simulink model "aircraft_pitch_lqr_multibody"  (R2022b)
settings: Solver=ode23t  StartTime=0.0  StopTime=stopTime  MaxStep=0.005  RelTol=1e-9  AbsTol=1e-11
model workspace (MAT data in the model file):
  Jpitch = 1
  K = [-0.5605 76.158 2.1817]
  Ki = 0
  Nbar = 2.1817
  aScale = 1
  biasAcceleration = 0
  biasStartTime = 30
  biasTime = 20
  deltaMax = 0.436332312999
  elevatorBias = 0
  geometryInertia = 4.77572166667
  integratorThreshold = 0.0174532925199
  massScale = 1
  r = 0.2
  stopTime = 30
undefined symbols (not defined in the file or in its folder): X, Y, Z
libraries: sm_lib x9, nesl_utility x4
settings Model: Creator=shark  LastModifiedBy=shark

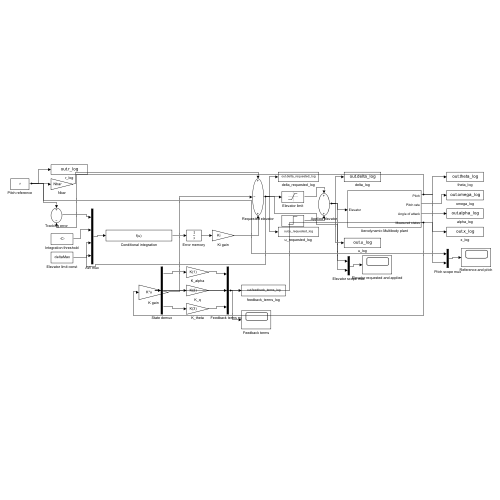
[thumbnail: Simulink's stored preview of the top-level diagram]
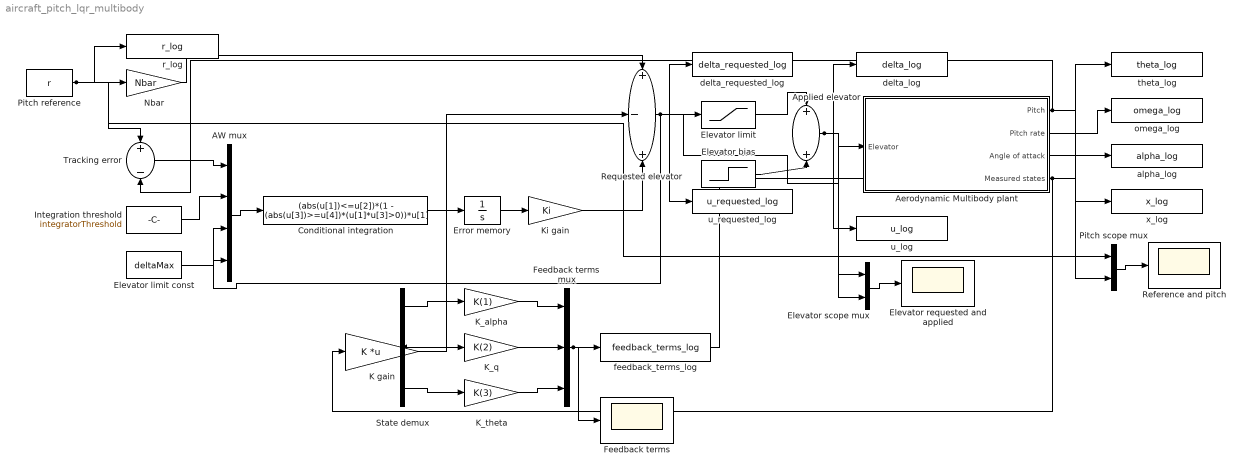
== system aircraft_pitch_lqr_multibody ==
  AW mux : Mux
  Aerodynamic Multibody plant : Subsystem
  Applied elevator : Sum
  Conditional integration : Fcn  Expr=(abs(u[1])<=u[2])*(1 - (abs(u[3])>=u[4])*(u[1]*u[3]>0))*u[1]
  Elevator bias : Step  Time=biasStartTime  After=elevatorBias  SampleTime=0
  Elevator limit : Saturate  UpperLimit=deltaMax  LowerLimit=-deltaMax
  Elevator limit const : Constant  Value=deltaMax
  Elevator requested and applied : Scope
  Elevator scope mux : Mux  Inputs=2
  Error memory : Integrator
  Feedback terms : Scope
  Feedback terms mux : Mux  Inputs=3
  Integration threshold : Constant  Value=integratorThreshold
  K gain : Gain  Gain=K  Multiplication=Matrix(K*u)
  K_alpha : Gain  Gain=K(1)
  K_q : Gain  Gain=K(2)
  K_theta : Gain  Gain=K(3)
  Ki gain : Gain  Gain=Ki
  Nbar : Gain  Gain=Nbar
  Pitch reference : Constant  Value=r
  Pitch scope mux : Mux  Inputs=2
  Reference and pitch : Scope
  Requested elevator : Sum  Inputs=+-+
  State demux : Demux  Outputs=3
  Tracking error : Sum  Inputs=+-
  alpha_log : ToWorkspace  VariableName=alpha_log  SaveFormat=Timeseries  SampleTime=-1
  delta_log : ToWorkspace  VariableName=delta_log  SaveFormat=Timeseries  SampleTime=-1
  delta_requested_log : ToWorkspace  VariableName=delta_requested_log  SaveFormat=Timeseries  SampleTime=-1
  feedback_terms_log : ToWorkspace  VariableName=feedback_terms_log  SaveFormat=Timeseries  SampleTime=-1
  omega_log : ToWorkspace  VariableName=omega_log  SaveFormat=Timeseries  SampleTime=-1
  r_log : ToWorkspace  VariableName=r_log  SaveFormat=Timeseries  SampleTime=-1
  theta_log : ToWorkspace  VariableName=theta_log  SaveFormat=Timeseries  SampleTime=-1
  u_log : ToWorkspace  VariableName=u_log  SaveFormat=Timeseries  SampleTime=-1
  u_requested_log : ToWorkspace  VariableName=u_requested_log  SaveFormat=Timeseries  SampleTime=-1
  x_log : ToWorkspace  VariableName=x_log  SaveFormat=Timeseries  SampleTime=-1
  wires:
  Pitch reference/1 -> Nbar/1, Tracking error/1, r_log/1, Pitch scope mux/1
  Aerodynamic Multibody plant/1(Pitch) -> Tracking error/2, theta_log/1, Pitch scope mux/2
  Tracking error/1 -> AW mux/1
  Integration threshold/1 -> AW mux/2
  Requested elevator/1 -> AW mux/3, Elevator limit/1, delta_requested_log/1, u_requested_log/1, Elevator scope mux/1
  Elevator limit const/1 -> AW mux/4
  AW mux/1 -> Conditional integration/1
  Conditional integration/1 -> Error memory/1
  Error memory/1 -> Ki gain/1
  Aerodynamic Multibody plant/4(Measured states) -> K gain/1, State demux/1, x_log/1
  State demux/1 -> K_alpha/1
  State demux/2 -> K_q/1
  State demux/3 -> K_theta/1
  K_alpha/1 -> Feedback terms mux/1
  K_q/1 -> Feedback terms mux/2
  K_theta/1 -> Feedback terms mux/3
  Nbar/1 -> Requested elevator/1
  K gain/1 -> Requested elevator/2
  Ki gain/1 -> Requested elevator/3
  Elevator limit/1 -> Applied elevator/1
  Elevator bias/1 -> Applied elevator/2
  Applied elevator/1 -> Aerodynamic Multibody plant/1(Elevator), delta_log/1, u_log/1, Elevator scope mux/2
  Aerodynamic Multibody plant/2(Pitch rate) -> omega_log/1
  Aerodynamic Multibody plant/3(Angle of attack) -> alpha_log/1
  Feedback terms mux/1 -> feedback_terms_log/1, Feedback terms/1
  Pitch scope mux/1 -> Reference and pitch/1
  Elevator scope mux/1 -> Elevator requested and applied/1

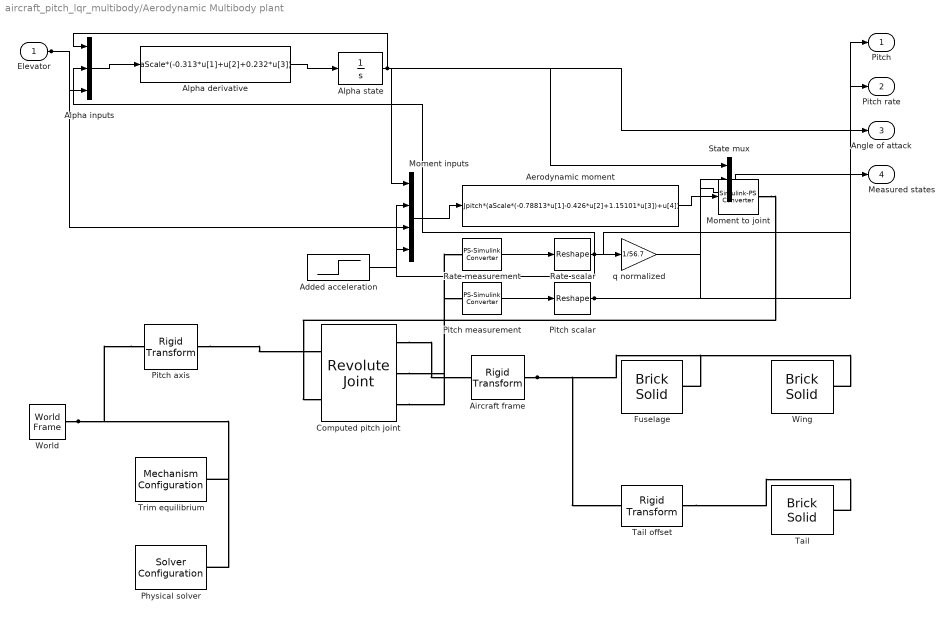
== system aircraft_pitch_lqr_multibody/Aerodynamic Multibody plant ==
  Elevator : Inport
  Added acceleration : Step  Time=biasTime  After=biasAcceleration  SampleTime=0
  Aerodynamic moment : Fcn  Expr=Jpitch*(aScale*(-0.78813*u[1]-0.426*u[2]+1.15101*u[3])+u[4])
  Aircraft frame : sm_lib/Frames and Transforms/Rigid Transform  TranslationMethod=None  TranslationStandardOffset=0  TranslationLengthUnit=m  TranslationStandardAxis=+Z  TranslationCartesianOffset=[0 0 0]  TranslationROffset=0  TranslationROffsetUnits=m  TranslationZOffset=0  TranslationZOffsetUnits=m  TranslationThetaOffset=0  TranslationThetaOffsetUnits=deg  RotationMethod=StandardAxis  RotationAngleUnits=deg  RotationStandardAxis=+X  RotationAngle=-90  RotationArbitraryAxis=[0 0 1]  FollAlignAxisA=+X  BaseAlignAxisA=+Y  FollAlignAxisB=+Y  BaseAlignAxisB=+Z  RotationSequenceAxes=FollowerAxes  RotationSequence=XYX  RotationSequenceAngles=[0 0 0]  RotationSequenceAnglesUnits=deg  RotationMatrix=[1 0 0; 0 1 0; 0 0 1]  Quaternion=[1 0 0 0]
  Alpha derivative : Fcn  Expr=aScale*(-0.313*u[1]+u[2]+0.232*u[3])
  Alpha inputs : Mux  Inputs=3
  Alpha state : Integrator
  Computed pitch joint : sm_lib/Joints/Revolute Joint  JointMode=Normal  SenseConstraintForce=off  SenseConstraintForceX=off  SenseConstraintForceY=off  SenseConstraintForceZ=off  SenseConstraintTorque=off  SenseConstraintTorqueX=off  SenseConstraintTorqueY=off  SenseConstraintTorqueZ=off  SenseTotalForce=off  SenseTotalForceX=off  SenseTotalForceY=off  SenseTotalForceZ=off  SenseTotalTorque=off  SenseTotalTorqueX=off  SenseTotalTorqueY=off  SenseTotalTorqueZ=off  CompositeWrenchDir=FollowerOnBase  CompositeWrenchFrame=BaseFrame  EquilibriumPosition=0  EquilibriumPositionUnits=deg  SpringStiffness=0  SpringStiffnessUnits=N*m/deg  DampingCoefficient=0  DampingCoefficientUnits=N*m/(deg/s)  TorqueActuationMode=InputTorque  MotionActuationMode=ComputedMotion  SensePosition=on  SenseVelocity=on  SenseAcceleration=off  SenseTorqueForce=off  SenseLowerLimitTorqueForce=off  SenseUpperLimitTorqueForce=off  LowerLimitSpecify=off  LowerLimitBound=-90  LowerLimitBoundUnits=deg  LowerLimitStiffness=1e4  LowerLimitStiffnessUnits=N*m/deg  LowerLimitDamping=10  LowerLimitDampingUnits=N*m/(deg/s)  LowerLimitTransitionRegionWidth=0.1  LowerLimitTransitionRegionWidthUnits=deg  UpperLimitSpecify=off  UpperLimitBound=90  UpperLimitBoundUnits=deg  UpperLimitStiffness=1e4  UpperLimitStiffnessUnits=N*m/deg  UpperLimitDamping=10  UpperLimitDampingUnits=N*m/(deg/s)  UpperLimitTransitionRegionWidth=0.1  UpperLimitTransitionRegionWidthUnits=deg  PositionTargetSpecify=on  PositionTargetPriority=High  PositionTargetValue=0  PositionTargetValueUnits=rad  VelocityTargetSpecify=on  VelocityTargetPriority=High  VelocityTargetValue=0  VelocityTargetValueUnits=rad/s
  Fuselage : sm_lib/Body Elements/Brick Solid  GraphicAmbientColor=[0.15 0.15 0.15 1.0]  BasedOnType=Mass  BrickDimensions=[8 .65 .65]  BrickDimensionUnits=m  CenterOfMass=[0 0 0]  CenterOfMassUnits=m  GraphicDiffuseColor=[.15 .45 .85]  Density=1000  DensityUnits=kg/m^3  DoExposeReferenceFrame=on  GraphicEmissiveColor=[0.0 0.0 0.0 1.0]  ExportEntireGeometry=off  SerializedFrames=<Frames/>  MarkerShape=Sphere  MarkerSize=10  GraphicType=FromGeometry  InertiaType=CalculateFromGeometry  Mass=.8*Jpitch/geometryInertia  MassUnits=kg  MomentsOfInertia=[1 1 1]  MomentsOfInertiaUnits=kg*m^2  GraphicOpacity=1.0  ProductsOfInertia=[0 0 0]  ProductsOfInertiaUnits=kg*m^2  GraphicShininess=75  GraphicSpecularColor=[0.5 0.5 0.5 1.0]  GraphicVisPropType=SimpleVisualProperties
  Moment inputs : Mux
  Moment to joint : nesl_utility/Simulink-PS Converter  PhysicalDomain=network_engine_domain  SubClassName=ps_input  LeftPortType=input  RightPortType=output  PseudoPeriodic=off  Frequencies=[]  NoiseDistribution=none  NoiseParameters=[]  Unit=N*m  AffineConversion=off  FilteringAndDerivatives=provide  SimscapeFilterOrder=1  InputFilterTimeConstant=0.001  UdotUserProvided=0
  Physical solver : nesl_utility/Solver Configuration  PhysicalDomain=network_engine_domain  SubClassName=solver  LeftPortType=input  RightPortType=generic  Tones=[]  Harmonics=[]  SimulateNoise=off  Profile=off  UseLocalSampling=off  EnableSwitchedLinearOptims=on  FrequencyDomain=off  UseCCode=off  RelTol=0.001  AbsTol=0.001  MinStep=1e-09  ToWorkspace=off  RevertToSquareIcSolve=off  NumHomotopyIterations=100  PhasorMode=off  PhasorModeNumHarmonics=1  ConsistencySolver=NEWTON_XTOL_AFTER_FTOL  IndexReductionMethod=DerivativeReplacement  DoDC=off  ResidualTolerance=1e-09  ConsistencyTolSource=GLOBAL  ConsistencyAbsTol=0.001  ConsistencyRelTol=0.001  ConsistencyTolFactor=0.001  UseLocalSolver=off  LocalSolverChoice=NE_BACKWARD_EULER_ADVANCER  ResolveIndetEquations=on  FunctionEvalNumThread=1  LocalSolverSampleTime=0.001  DoFixedCost=off  MaxNonlinIter=3  MaxModeIter=2  ComputeImpulses=off  ImpulseIterations=2  LinearAlgebra=auto  LinearAlgebraNumThread=0  EquationFormulation=NE_TIME_EF  DelaysMemoryBudget=1024  AutomaticFiltering=on  FilteringTimeConstant=0.001  PartitionStorageMethod=AS_NEEDED  PartitionMemoryBudget=1024  PartitionMethod=ROBUST
  Pitch axis : sm_lib/Frames and Transforms/Rigid Transform  TranslationMethod=None  TranslationStandardOffset=0  TranslationLengthUnit=m  TranslationStandardAxis=+Z  TranslationCartesianOffset=[0 0 0]  TranslationROffset=0  TranslationROffsetUnits=m  TranslationZOffset=0  TranslationZOffsetUnits=m  TranslationThetaOffset=0  TranslationThetaOffsetUnits=deg  RotationMethod=StandardAxis  RotationAngleUnits=deg  RotationStandardAxis=+X  RotationAngle=90  RotationArbitraryAxis=[0 0 1]  FollAlignAxisA=+X  BaseAlignAxisA=+Y  FollAlignAxisB=+Y  BaseAlignAxisB=+Z  RotationSequenceAxes=FollowerAxes  RotationSequence=XYX  RotationSequenceAngles=[0 0 0]  RotationSequenceAnglesUnits=deg  RotationMatrix=[1 0 0; 0 1 0; 0 0 1]  Quaternion=[1 0 0 0]
  Pitch measurement : nesl_utility/PS-Simulink Converter  PhysicalDomain=network_engine_domain  SubClassName=ps_output  LeftPortType=input  RightPortType=output  PseudoPeriodic=off  Frequencies=[]  VectorFormat=inherit  Unit=rad  AffineConversion=off
  Pitch scalar : Reshape
  Rate measurement : nesl_utility/PS-Simulink Converter  PhysicalDomain=network_engine_domain  SubClassName=ps_output  LeftPortType=input  RightPortType=output  PseudoPeriodic=off  Frequencies=[]  VectorFormat=inherit  Unit=rad/s  AffineConversion=off
  Rate scalar : Reshape
  State mux : Mux  Inputs=3
  Tail : sm_lib/Body Elements/Brick Solid  GraphicAmbientColor=[0.15 0.15 0.15 1.0]  BasedOnType=Mass  BrickDimensions=[1 3 .1]  BrickDimensionUnits=m  CenterOfMass=[0 0 0]  CenterOfMassUnits=m  GraphicDiffuseColor=[.3 .55 .85]  Density=1000  DensityUnits=kg/m^3  DoExposeReferenceFrame=on  GraphicEmissiveColor=[0.0 0.0 0.0 1.0]  ExportEntireGeometry=off  SerializedFrames=<Frames/>  MarkerShape=Sphere  MarkerSize=10  GraphicType=FromGeometry  InertiaType=CalculateFromGeometry  Mass=.05*Jpitch/geometryInertia  MassUnits=kg  MomentsOfInertia=[1 1 1]  MomentsOfInertiaUnits=kg*m^2  GraphicOpacity=1.0  ProductsOfInertia=[0 0 0]  ProductsOfInertiaUnits=kg*m^2  GraphicShininess=75  GraphicSpecularColor=[0.5 0.5 0.5 1.0]  GraphicVisPropType=SimpleVisualProperties
  Tail offset : sm_lib/Frames and Transforms/Rigid Transform  TranslationMethod=Cartesian  TranslationStandardOffset=0  TranslationLengthUnit=m  TranslationStandardAxis=+Z  TranslationCartesianOffset=[-3 0 .2]  TranslationROffset=0  TranslationROffsetUnits=m  TranslationZOffset=0  TranslationZOffsetUnits=m  TranslationThetaOffset=0  TranslationThetaOffsetUnits=deg  RotationMethod=None  RotationAngleUnits=deg  RotationStandardAxis=+Z  RotationAngle=0.0  RotationArbitraryAxis=[0 0 1]  FollAlignAxisA=+X  BaseAlignAxisA=+Y  FollAlignAxisB=+Y  BaseAlignAxisB=+Z  RotationSequenceAxes=FollowerAxes  RotationSequence=XYX  RotationSequenceAngles=[0 0 0]  RotationSequenceAnglesUnits=deg  RotationMatrix=[1 0 0; 0 1 0; 0 0 1]  Quaternion=[1 0 0 0]
  Trim equilibrium : sm_lib/Utilities/Mechanism Configuration  UniformGravity=Constant  GravityVector=[0 0 0]  GravityUnits=m/s^2  LinearizationDelta=0.001  JointModeTransitionNonlinearIterations=2
  Wing : sm_lib/Body Elements/Brick Solid  GraphicAmbientColor=[0.15 0.15 0.15 1.0]  BasedOnType=Mass  BrickDimensions=[1.4 8 .12]  BrickDimensionUnits=m  CenterOfMass=[0 0 0]  CenterOfMassUnits=m  GraphicDiffuseColor=[.65 .75 .9]  Density=1000  DensityUnits=kg/m^3  DoExposeReferenceFrame=on  GraphicEmissiveColor=[0.0 0.0 0.0 1.0]  ExportEntireGeometry=off  SerializedFrames=<Frames/>  MarkerShape=Sphere  MarkerSize=10  GraphicType=FromGeometry  InertiaType=CalculateFromGeometry  Mass=.15*Jpitch/geometryInertia  MassUnits=kg  MomentsOfInertia=[1 1 1]  MomentsOfInertiaUnits=kg*m^2  GraphicOpacity=1.0  ProductsOfInertia=[0 0 0]  ProductsOfInertiaUnits=kg*m^2  GraphicShininess=75  GraphicSpecularColor=[0.5 0.5 0.5 1.0]  GraphicVisPropType=SimpleVisualProperties
  World : sm_lib/Frames and Transforms/World Frame
  q normalized : Gain  Gain=1/56.7
  Pitch : Outport
  Pitch rate : Outport  Port=2
  Angle of attack : Outport  Port=3
  Measured states : Outport  Port=4
  wires:
  Alpha state/1 -> Alpha inputs/1, Moment inputs/1, State mux/1, Angle of attack/1
  Rate scalar/1 -> Alpha inputs/2, Moment inputs/2, q normalized/1, Pitch rate/1
  Elevator/1 -> Alpha inputs/3, Moment inputs/3
  Alpha inputs/1 -> Alpha derivative/1
  Alpha derivative/1 -> Alpha state/1
  Added acceleration/1 -> Moment inputs/4
  Moment inputs/1 -> Aerodynamic moment/1
  Aerodynamic moment/1 -> Moment to joint/1
  Pitch measurement/1 -> Pitch scalar/1
  Rate measurement/1 -> Rate scalar/1
  q normalized/1 -> State mux/2
  Pitch scalar/1 -> State mux/3, Pitch/1
  State mux/1 -> Measured states/1
  connections:
  Pitch axis/LConn1 -- World/RConn1 -- Trim equilibrium/RConn1 -- Physical solver/RConn1
  Pitch axis/RConn1 -- Computed pitch joint/LConn1
  Moment to joint/RConn1 -- Computed pitch joint/LConn2
  Computed pitch joint/RConn1 -- Aircraft frame/LConn1
  Computed pitch joint/RConn2 -- Pitch measurement/LConn1
  Computed pitch joint/RConn3 -- Rate measurement/LConn1
  Fuselage/RConn1 -- Aircraft frame/RConn1 -- Wing/RConn1 -- Tail offset/LConn1
  Tail offset/RConn1 -- Tail/RConn1
